simulink model "road"  (R2018b)
settings: Solver=VariableStepAuto  StartTime=0.0  StopTime=10.0  RelTol=1e-3
libraries: fuzblock x2, simulink x2
settings Model: Creator=Nick  LastModifiedBy=Nick

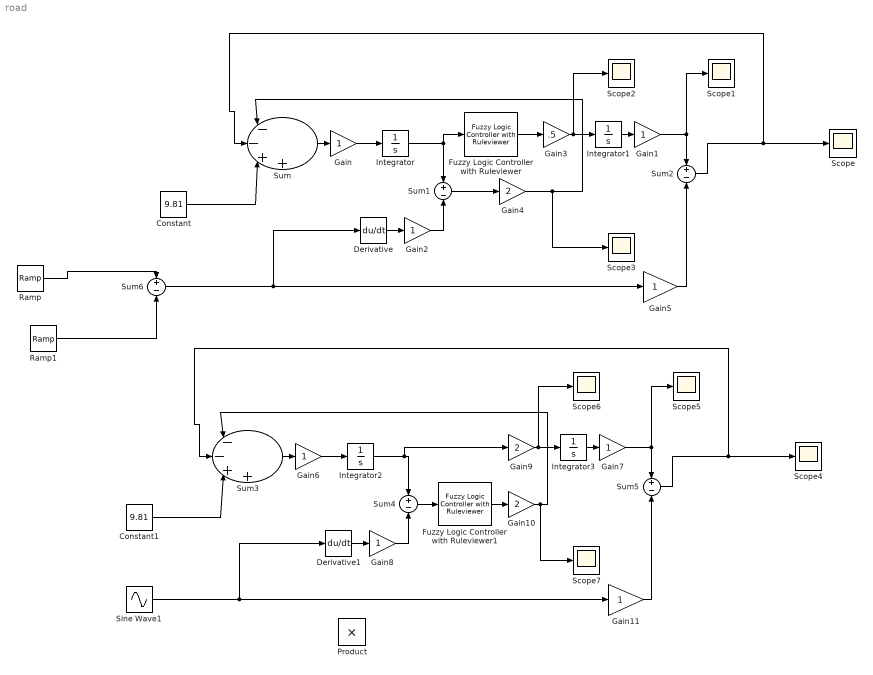
== system road ==
  Constant : Constant  Value=9.81
  Constant1 : Constant  Value=9.81
  Derivative : Derivative
  Derivative1 : Derivative
  Fuzzy Logic Controller with Ruleviewer : fuzblock/Fuzzy Logic  Controller  with Ruleviewer  fismatrix=fuzzyroad1  Ts=2
  Fuzzy Logic Controller with Ruleviewer1 : fuzblock/Fuzzy Logic  Controller  with Ruleviewer  fismatrix=fuzzyroad1  Ts=2
  Gain{,1..2,5..8,11} (8 alike) : Gain
  Gain10 : Gain  Gain=2
  Gain3 : Gain  Gain=.5
  Gain4 : Gain  Gain=2
  Gain9 : Gain  Gain=2
  Integrator{,1..3} (4 alike) : Integrator
  Product : Product
  Ramp : simulink/Sources/Ramp  slope=1  start=0  InitialOutput=0
  Ramp1 : simulink/Sources/Ramp  slope=-1  start=2  InitialOutput=0
  Scope{,1..7} (8 alike) : Scope
  Sine Wave1 : Sin  Amplitude=.5  SampleTime=0
  Sum : Sum  Inputs=|--++
  Sum{1..2,4..6} (5 alike) : Sum  Inputs=+-
  Sum3 : Sum  Inputs=|--++
  wires:
  Sum/1 -> Gain/1
  Sum1/1 -> Gain4/1
  Integrator1/1 -> Gain1/1
  Constant/1 -> Sum/3
  Derivative/1 -> Gain2/1
  Sum2/1 -> Scope/1, Sum/2
  Gain1/1 -> Scope1/1, Sum2/1
  Gain/1 -> Integrator/1
  Gain2/1 -> Sum1/2
  Gain4/1 -> Scope3/1, Sum/1
  Sum6/1 -> Gain5/1, Derivative/1
  Gain5/1 -> Sum2/2
  Integrator/1 -> Fuzzy Logic Controller with Ruleviewer/1, Sum1/1
  Gain3/1 -> Scope2/1, Integrator1/1
  Fuzzy Logic Controller with Ruleviewer/1 -> Gain3/1
  Sine Wave1/1 -> Gain11/1, Derivative1/1
  Gain10/1 -> Scope7/1, Sum3/1
  Gain8/1 -> Sum4/2
  Gain7/1 -> Scope5/1, Sum5/1
  Sum4/1 -> Fuzzy Logic Controller with Ruleviewer1/1
  Integrator3/1 -> Gain7/1
  Sum3/1 -> Gain6/1
  Derivative1/1 -> Gain8/1
  Constant1/1 -> Sum3/3
  Gain6/1 -> Integrator2/1
  Gain9/1 -> Scope6/1, Integrator3/1
  Gain11/1 -> Sum5/2
  Sum5/1 -> Scope4/1, Sum3/2
  Integrator2/1 -> Gain9/1, Sum4/1
  Fuzzy Logic Controller with Ruleviewer1/1 -> Gain10/1
  Ramp1/1 -> Sum6/2
  Ramp/1 -> Sum6/1
